simulink model "difference_eq"  (R2020a)
settings: Solver=VariableStepAuto  StartTime=0.0  StopTime=10.0  RelTol=1e-3
settings Model: Creator=kolep  LastModifiedBy=kolep

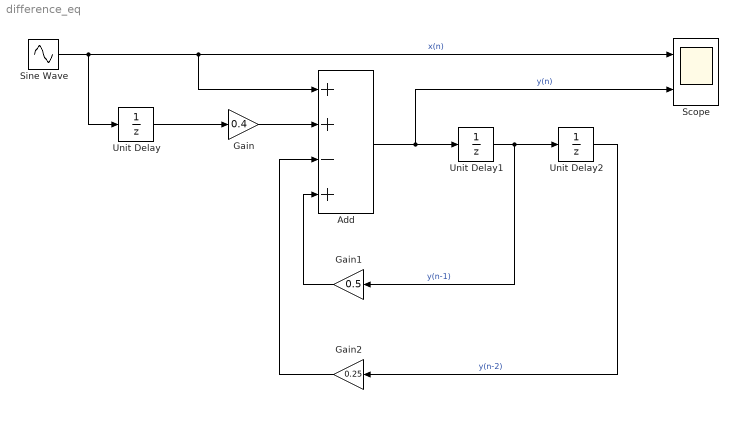
== system difference_eq ==
  Add : Sum  Inputs=++-+
  Gain : Gain  Gain=0.4
  Gain1 : Gain  Gain=0.5
  Gain2 : Gain  Gain=0.25
  Scope : Scope  NumInputPorts=2
  Sine Wave : Sin  SampleTime=0
  Unit Delay : UnitDelay  SampleTime=-1  HasFrameUpgradeWarning=on
  Unit Delay1 : UnitDelay  SampleTime=-1  HasFrameUpgradeWarning=on
  Unit Delay2 : UnitDelay  SampleTime=-1  HasFrameUpgradeWarning=on
  wires:
  Sine Wave/1 -> Unit Delay/1, Add/1, Scope/1  "x(n)"
  Gain/1 -> Add/2
  Unit Delay/1 -> Gain/1
  Add/1 -> Scope/2, Unit Delay1/1  "y(n)"
  Unit Delay1/1 -> Gain1/1, Unit Delay2/1  "y(n-1)"
  Unit Delay2/1 -> Gain2/1  "y(n-2)"
  Gain1/1 -> Add/4
  Gain2/1 -> Add/3
